simulink model "c_proje_sim"  (R2020b)
settings: Solver=VariableStepAuto  StartTime=0.0  StopTime=100  RelTol=1e-3
libraries: simulink x1
settings Model: Creator=musa oğural  LastModifiedBy=musa oğural

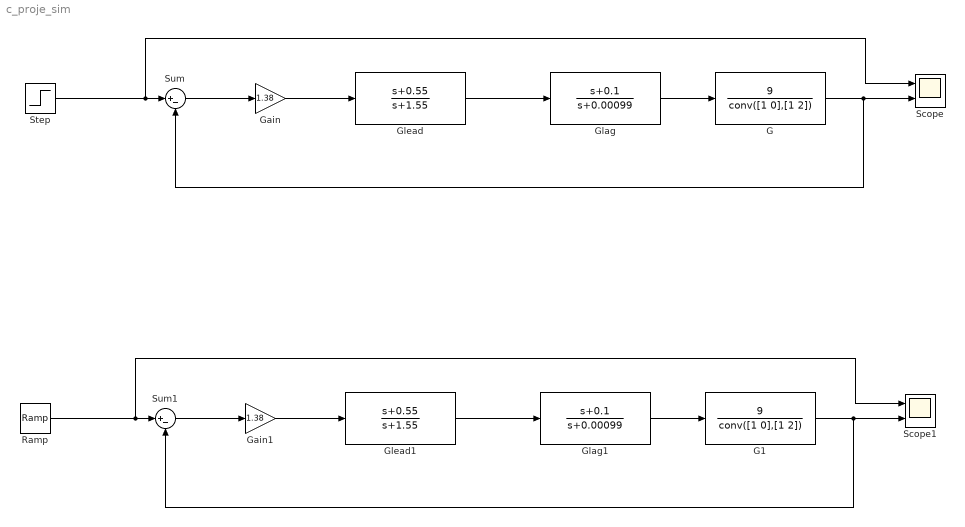
== system c_proje_sim ==
  G : TransferFcn  Numerator=[9]  Denominator=conv([1 0],[1 2])
  G1 : TransferFcn  Numerator=[9]  Denominator=conv([1 0],[1 2])
  Gain : Gain  Gain=1.38
  Gain1 : Gain  Gain=1.38
  Glag : TransferFcn  Numerator=[1 0.1]  Denominator=[1 0.00099]
  Glag1 : TransferFcn  Numerator=[1 0.1]  Denominator=[1 0.00099]
  Glead : TransferFcn  Numerator=[1 0.55]  Denominator=[1 1.55]
  Glead1 : TransferFcn  Numerator=[1 0.55]  Denominator=[1 1.55]
  Ramp : simulink/Sources/Ramp  slope=1  start=0  InitialOutput=0
  Scope : Scope  NumInputPorts=2
  Scope1 : Scope  NumInputPorts=2
  Step : Step  Time=0  SampleTime=0
  Sum : Sum  Inputs=|+-
  Sum1 : Sum  Inputs=|+-
  wires:
  Sum/1 -> Gain/1
  Glead/1 -> Glag/1
  Gain/1 -> Glead/1
  Step/1 -> Scope/1, Sum/1
  Glag/1 -> G/1
  G/1 -> Sum/2, Scope/2
  Glag1/1 -> G1/1
  Ramp/1 -> Scope1/1, Sum1/1
  G1/1 -> Sum1/2, Scope1/2
  Gain1/1 -> Glead1/1
  Sum1/1 -> Gain1/1
  Glead1/1 -> Glag1/1
